simulink model "combiner_test"  (R2021b)
settings: Solver=VariableStepAuto  StartTime=0.0  StopTime=stop_time-1  RelTol=1e-3
libraries: dspsrcs4 x2
settings Model: Creator=torha  LastModifiedBy=torha

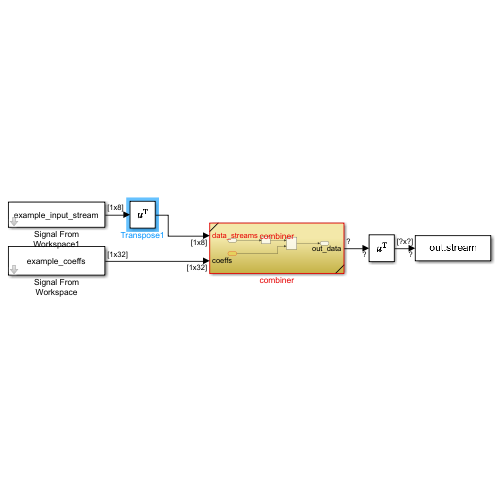
[thumbnail: Simulink's stored preview of the top-level diagram]
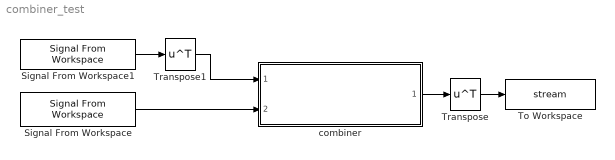
== system combiner_test ==
  Signal From Workspace : dspsrcs4/Signal From Workspace  X=example_coeffs  Ts=1  nsamps=1  OutputAfterFinalValue=Setting to zero  ignoreOrWarnInputAndFrameLengths=off  OutputFrames=off
  Signal From Workspace1 : dspsrcs4/Signal From Workspace  X=example_input_stream  Ts=1  nsamps=1  OutputAfterFinalValue=Setting to zero  ignoreOrWarnInputAndFrameLengths=off  OutputFrames=off
  To Workspace : ToWorkspace  VariableName=stream  SampleTime=-1
      settings: Save2DSignal=2-D array (concatenate along first dimension)
  Transpose : Math  Operator=transpose  SaturateOnIntegerOverflow=on
  Transpose1 : Math  Operator=transpose  SaturateOnIntegerOverflow=on
  combiner : Subsystem  ReferencedSubsystem=combiner
  wires:
  Signal From Workspace1/1 -> Transpose1/1
  combiner/1 -> Transpose/1
  Signal From Workspace/1 -> combiner/2
  Transpose/1 -> To Workspace/1
  Transpose1/1 -> combiner/1
